simulink model "Driver_Glider"  (R2022b)
settings: Solver=ode45  StartTime=0.0  StopTime=StopTime  FixedStep=1e-4  MaxStep=0.1  RelTol=1e-3  EnableMultiTasking=on
PostLoadFcn:
  | GliderDir = pwd;
  | 
  | cd ..\;
  | SimulinkDir = pwd;
  | addpath(SimulinkDir);
  | 
  | cd(GliderDir);
model workspace (MAT data in the model file):
  DrCycles.C505 = [0 1 2 3 4 5 6 7 8 9 10 11 ... (1012 elements, 506x2)]
  DrCycles.FTP = [0 1 2 3 4 5 6 7 8 9 10 11 ... (4956 elements, 2478x2)]
  DrCycles.UDDS = [0 1 2 3 4 5 6 7 8 9 10 11 ... (2746 elements, 1373x2)]
  DrCycles.HWFET = [0 1 2 3 4 5 6 7 8 9 10 11 ... (1532 elements, 766x2)]
  DrCycles.US06 = [0 1 2 3 4 5 6 7 8 9 10 11 ... (1194 elements, 597x2)]
  DrCycles.US06City = [0 1 2 3 4 5 6 7 8 9 10 11 ... (466 elements, 233x2)]
  DrCycles.US06Hwy = [0 1 2 3 4 5 6 7 8 9 10 11 ... (742 elements, 371x2)]
  DriverPic = [255 255 255 255 255 255 255 255 255 255 255 255 ... (1049040 elements, 940x372x3)]
  TimeHWFET = 765
  TimeUDDS = 1372
  TimeUS06 = 596
  VehiclePic = [252 252 252 252 252 252 252 252 252 252 252 252 ... (1047540 elements, 316x1105x3)]
  aeroDragCoeff = 0.38
  airDensity = 1.23
  frontArea = 2.1
  gravity = 9.81
  inclinationAngle = 0
  inertialMassVeh = 2392
  massVeh = 2300
  rollingResistCoeff = 0.01
values from neighbouring files (symbols this model uses):
  D_Driver = 0    [Driver_Glider_Params.m]
  GR = Ndriven/Ndriving    (= 3)    [Driver_Glider_Params.m]
  I_Driver = 1    [Driver_Glider_Params.m]
  P_Driver = 250    [Driver_Glider_Params.m]
  r_wheel = .254    (= 0.254)    [Driver_Glider_Params.m]
  time_step = time(2)    [Driver_Glider_Params.m]
  tractiveForceMax = torqueMax*GR/r_wheel    (= 177.165354331)    [Driver_Glider_Params.m]
undefined symbols (not defined in the file or in its folder): magnitude
libraries: slpidlib x1
(part 1 of 2)
CloseFcn:
  | rmpath(SimulinkDir);
  | clear GliderDir SimulinkDir;
settings Model: Creator=EduardoMarquez  LastModifiedBy=skylarlennon
settings SolverCC: AlgebraicLoopSolver=TrustRegion
settings DataIOCC: ExternalInput=[US06]  LimitDataPoints=on  SaveFormat=Array  SignalLoggingSaveFormat=ModelDataLogs  ReturnWorkspaceOutputs=off
settings OptimizationCC: LifeSpan=inf
settings DebuggingCC: SolverPrmCheckMsg=warning  UnconnectedInputMsg=warning  UnconnectedOutputMsg=warning  UnconnectedLineMsg=warning  SFUnexpectedBacktrackingDiag=warning  SFNoUnconditionalDefaultTransitionDiag=warning  SFExecutionAtInitializationDiag=none  SFMachineParentedDataDiag=warning  ArithmeticOperatorsInVariantConditions=warning
settings HardwareCC: ProdBitPerPointer=32  ProdBitPerSizeT=32  ProdBitPerPtrDiffT=32  ProdLargestAtomicFloat=None  ProdIntDivRoundTo=Undefined  ProdEndianess=Unspecified  ProdWordSize=32  ProdHWDeviceType=32-bit Generic
settings ModelReferenceCC: EnableRefExpFcnMdlSchedulingChecks=on  PropagateSignalLabelsOutOfModel=off
settings SFSimCC: SimUseLocalCustomCode=off  CustomCodeUndefinedFunction=UseInterfaceOnly
settings RTWCC: RTWUseLocalCustomCode=off
settings CodeAppCC: StateflowObjectComments=on
settings GRTTargetCC: TargetLangStandard=C89/C90 (ANSI)
settings ConfigComp: CovMetricSettings=dw  CovSaveCumulativeToWorkspaceVar=on  CovSaveSingleToWorkspaceVar=on  CovExternalEMLEnable=off  CovSFcnEnable=off

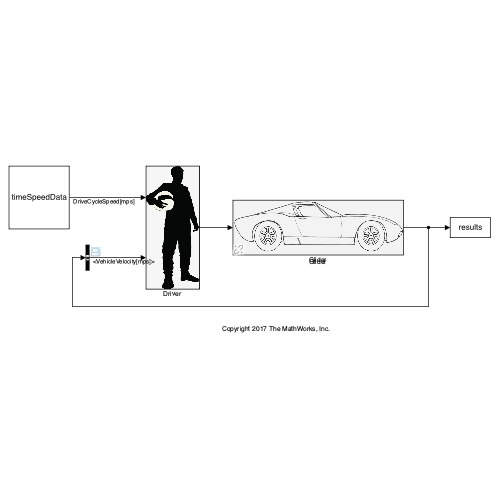
[thumbnail: Simulink's stored preview of the top-level diagram]
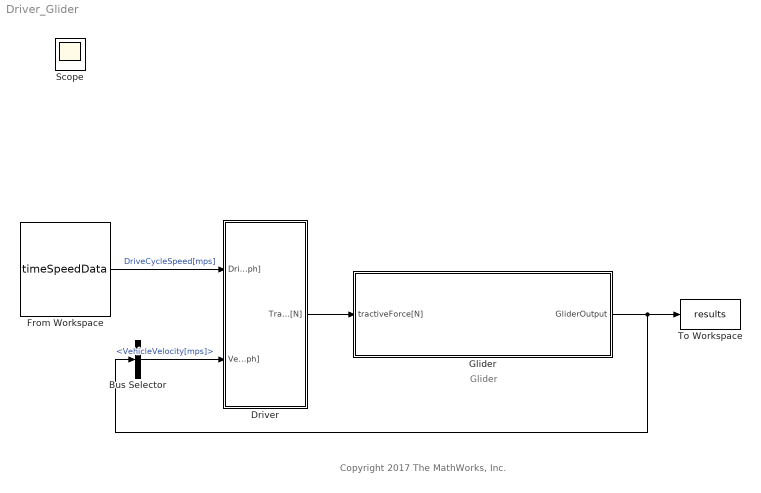
== system Driver_Glider ==
  note: Glider
  note: Copyright 2017 The MathWorks, Inc.
  Bus Selector : BusSelector  OutputSignals=VehicleVelocity[mps]
  Driver : Subsystem
      mask Display: image('$imagefile'); % Use "Edit Image" on toolstrip to change.
  From Workspace : FromWorkspace  VariableName=timeSpeedData  SampleTime=time_step
  Glider : Subsystem  AncestorBlock=Driver_Glider_Library/Glider
      mask Display: image('$imagefile'); % Use "Edit Image" on toolstrip to change.
  To Workspace : ToWorkspace  VariableName=results  SampleTime=-1
  Scope : Scope
  wires:
  From Workspace/1 -> Driver/1(DriveCycleSpeed[mph])  "DriveCycleSpeed[mps]"
  Driver/1(TractiveForce[N]) -> Glider/1(tractiveForce[N])
  Glider/1(GliderOutput) -> To Workspace/1, Bus Selector/1
  Bus Selector/1 -> Driver/2(VehicleSpeed[mph])  "<VehicleVelocity[mps]>"
